simulink model "start_PLL_2018b"  (R2018b)
settings: Solver=FixedStepAuto  StartTime=0.0  StopTime=inf  RelTol=1e-3
undefined symbols (not defined in the file or in its folder): DiscIntNeverNeededParam
libraries: commfilt2 x2, commdigbbndam3 x2, commchan3 x1, commrandsrc3 x1, commsync2 x1, commsink2 x1, commrflib2 x1
settings Model: Creator=Federal_PC  LastModifiedBy=Federal_PC
settings DataIOCC: ReturnWorkspaceOutputs=on
settings DebuggingCC: SFMachineParentedDataDiag=error

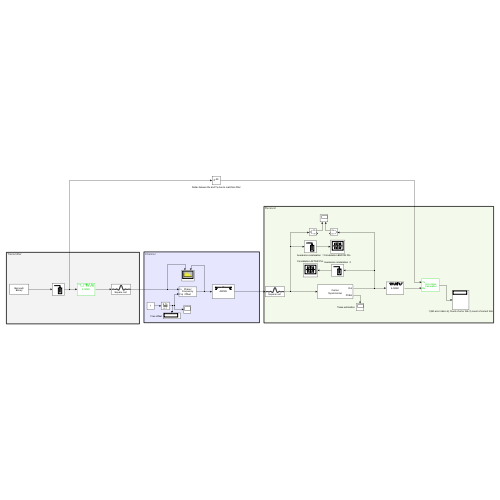
[thumbnail: Simulink's stored preview of the top-level diagram]
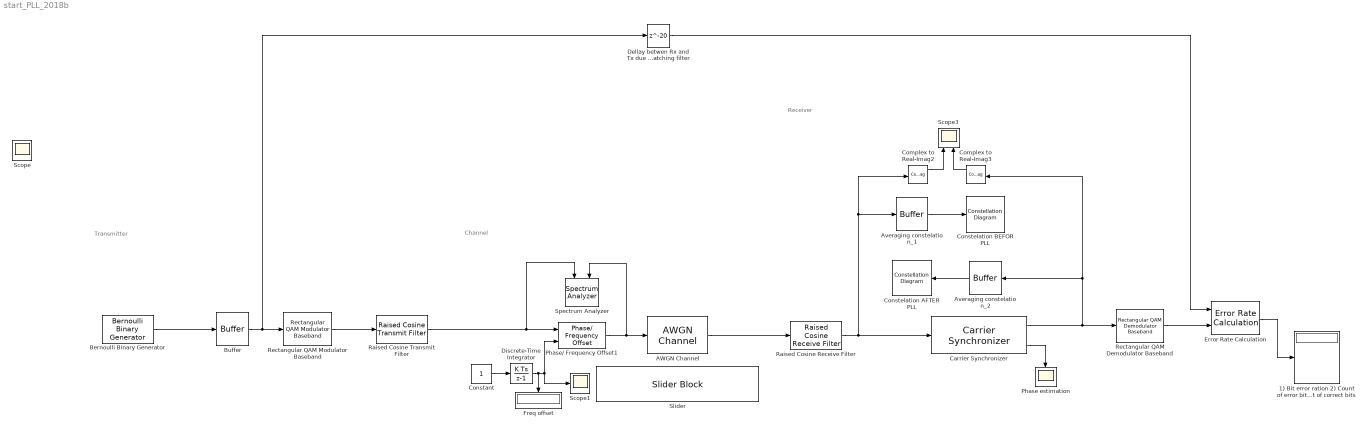
== system start_PLL_2018b ==
  note: Receiver
  note: Transmitter
  note: Channel
  1) Bit error ration 2) Count of error bits 3) count of correct bits : Display
  AWGN Channel : commchan3/AWGN Channel  InputProcessing=Columns as channels (frame based)  seed=67  noiseMode="Signal to noise ratio  (SNR)"  EbNodB=15  EsNodB=10  SNRdB=30  bitsPerSym=1  Ps=1  Tsym=1  variance=1
  Averaging constelation_1 : Buffer  N=100  OutputFrames=off
  Averaging constelation_2 : Buffer  N=100  OutputFrames=off
  Bernoulli Binary Generator : commrandsrc3/Bernoulli Binary Generator  ProbabilityOfZero=0.5  SeedSource=Auto  Seed=0  SampleTime=(1/200e3)/2  SamplesPerFrame=1  OutputDataType=double  SimulateUsing=Interpreted execution
  Buffer : Buffer  N=2  OutputFrames=off
  Carrier Synchronizer : commsync2/Carrier Synchronizer  Modulation=QAM  ModulationPhaseOffset=Auto  CustomPhaseOffset=0  SamplesPerSymbol=4  DampingFactor=0.707  NormalizedLoopBandwidth=0.01  EstimatedPhaseErrorOutputPort=on  SimulateUsing=Code generation
  Complex to Real-Imag2 : ComplexToRealImag
  Complex to Real-Imag3 : ComplexToRealImag
  Constant : Constant  SampleTime=1/100
  Constelation AFTER PLL : ConstellationDiagram
  Constelation BEFOR PLL : ConstellationDiagram
  Dellay betwen Rx and Tx due to matching filter : Delay  DelayLength=20
  Discrete-Time Integrator : DiscreteIntegrator  gainval=10e2  SampleTime=-1  ICPrevOutput=DiscIntNeverNeededParam  ICPrevScaledInput=DiscIntNeverNeededParam
  Error Rate Calculation : commsink2/Error Rate Calculation  N=0  st_delay=0  cp_mode=Entire frame  subframe=[]  PMode=Port  WsName=ErrorVec  RsMode2=off  stop=off  numErr=100  maxBits=1e6
  Freq offset : Display
  Phase estimation : Scope
  Phase/ Frequency Offset1 : commrflib2/Phase// Frequency Offset  phaseOffset=0  freqPort=on  freqOffset=3
  Raised Cosine Receive Filter : commfilt2/Raised Cosine Receive Filter  filtType=Square root  R=0.2  filtSpan=20  N=4  downFactor=4  downOffset=0  filterGain=1  RateOptions=Allow multirate processing  framing=Mute  checkCoeff=off  variableName=rcRxFilt  currentFiltSpan=10  D=5  inputOffset=0  sampMode=Mute  saveAsFlag=0  rateMode=Downsampling  checkGain=Normalized  launchFVT=on  roundingMode=Floor  overflowMode=off  coeffDataTypeStr=Inherit: Same word length as input  coeffMin=[]  coeffMax=[]  coeffLastDataTypeStr=Inherit: Same word length as input  accumDataTypeStr=Inherit: Same as product output  accumLastDataTypeStr=Inherit: Same as product output  outputDataTypeStr=Inherit: Same as accumulator  outputMin=[]  outputMax=[]  outputLastDataTypeStr=Inherit: Same as accumulator
  Raised Cosine Transmit Filter : commfilt2/Raised Cosine Transmit Filter  filtType=Square root  R=0.2  filtSpan=20  N=4  filterGain=1  RateOptions=Allow multirate processing  framing=Mute  checkCoeff=off  variableName=rcTxFilt  checkGain=Normalized  sampMode=Mute  saveAsFlag=0  currentFiltSpan=10  D=5  launchFVT=on  roundingMode=Floor  overflowMode=off  coeffDataTypeStr=Inherit: Same word length as input  coeffMin=[]  coeffMax=[]  coeffLastDataTypeStr=Inherit: Same word length as input  outputDataTypeStr=Inherit: Same as accumulator  outputMin=[]  outputMax=[]  outputLastDataTypeStr=Inherit: Same as accumulator
  Rectangular QAM Demodulator Baseband : commdigbbndam3/Rectangular QAM Demodulator Baseband  M=4  OutType=Bit  DecType=Hard decision  VarSource=Dialog  Variance=1  Dec=Gray  Mapping=[0:15]  PowType=Min. distance between symbols  MinDist=2  AvgPow=1  PeakPow=1  Ph=0  outDtype1=Inherit via internal rule  outDtype2=Inherit via internal rule  derotateFactorWordLen=16  derotateFactorDataTypeStr=Inherit: Same word length as input  derotateFactorLastDataTypeStr=Inherit: Same word length as input  denormFactorWordLen=16  denormFactorDataTypeStr=Inherit: Same word length as input  denormFactorLastDataTypeStr=Inherit: Same word length as input  prodOutWordLen=32  prodOutOverflowMode=Wrap  prodOutRoundingMode=Floor  prodOutOvFlMode=off  prodOutOvFlModeLastStrValue=off  sumWordLen=32
  Rectangular QAM Modulator Baseband : commdigbbndam3/Rectangular QAM Modulator Baseband  M=4  InType=Bit  Enc=Gray  Mapping=[0:15]  PowType=Min. distance between symbols  MinDist=2  AvgPow=1  PeakPow=1  Ph=0  outDtype=double  outWordLen=16  outUDDataType=sfix(16)  outFracLenMode=Best precision  outFracLen=15  outDataTypeStr=double  outLastDataTypeStr=double
  Scope1 : Scope
  Scope3 : Scope  NumInputPorts=2
  Slider : SliderBlock  ScaleMin=-10  ScaleMax=30  TickInterval=5  WebBlockId=24
  Spectrum Analyzer : SpectrumAnalyzer  NumInputPorts=2
  Scope : Scope
  wires:
  Bernoulli Binary Generator/1 -> Buffer/1
  Buffer/1 -> Dellay betwen Rx and Tx due to matching filter/1, Rectangular QAM Modulator Baseband/1
  Rectangular QAM Modulator Baseband/1 -> Raised Cosine Transmit Filter/1
  Raised Cosine Transmit Filter/1 -> Spectrum Analyzer/1, Phase/ Frequency Offset1/1
  Error Rate Calculation/1 -> 1) Bit error ration 2) Count of error bits 3) count of correct bits/1
  Dellay betwen Rx and Tx due to matching filter/1 -> Error Rate Calculation/1
  Rectangular QAM Demodulator Baseband/1 -> Error Rate Calculation/2
  Discrete-Time Integrator/1 -> Scope1/1, Phase/ Frequency Offset1/2, Freq offset/1
  Constant/1 -> Discrete-Time Integrator/1
  Phase/ Frequency Offset1/1 -> Spectrum Analyzer/2, AWGN Channel/1
  Complex to Real-Imag2/1 -> Scope3/1
  Complex to Real-Imag3/1 -> Scope3/2
  Raised Cosine Receive Filter/1 -> Carrier Synchronizer/1, Complex to Real-Imag2/1, Averaging constelation_1/1
  Averaging constelation_2/1 -> Constelation AFTER PLL/1
  AWGN Channel/1 -> Raised Cosine Receive Filter/1
  Carrier Synchronizer/1 -> Rectangular QAM Demodulator Baseband/1, Complex to Real-Imag3/1, Averaging constelation_2/1
  Carrier Synchronizer/2 -> Phase estimation/1
  Averaging constelation_1/1 -> Constelation BEFOR PLL/1
